simulink model "Solar_position_model"  (R2024a)
settings: Solver=VariableStepAuto  StartTime=0.0  StopTime=5  RelTol=1e-3
Description:
  | Acccurate Solar positioning algorithm
settings Model: Creator=Asus  LastModifiedBy=Asus

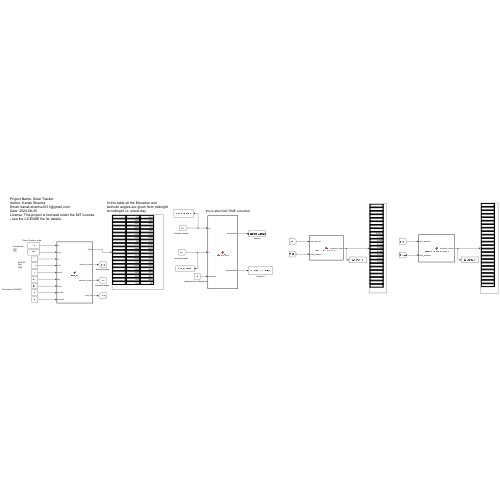
[thumbnail: Simulink's stored preview of the top-level diagram]
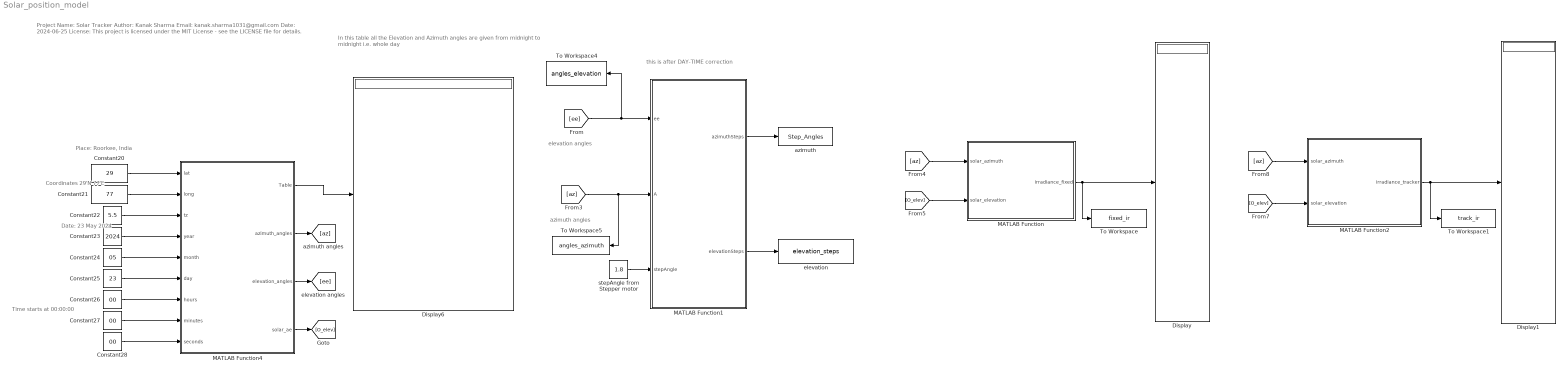
== system Solar_position_model ==
  note: Project Name: Solar Tracker
      | Author: Kanak Sharma
      | Email: kanak.sharma1031@gmail.com
      | Date: 2024-06-25
      | License: This project is licensed under the MIT License - see the LICENSE file for details.
  note: elevation angles
  note: In this table all the Elevation and Azimuth angles are given from midnight to midnight i.e. whole day
  note: Time starts at 00:00:00
  note: Coordinates
      | 29'N
      | 77'E
  note: azimuth angles
  note: this is after DAY-TIME correction
  note: Date: 23 May 2024
  note: Place: Roorkee, India
  Constant20 : Constant  Value=29
  Constant21 : Constant  Value=77
  Constant22 : Constant  Value=5.5
  Constant23 : Constant  Value=2024
  Constant24 : Constant  Value=05
  Constant25 : Constant  Value=23
  Constant26 : Constant  Value=00
  Constant27 : Constant  Value=00
  Constant28 : Constant  Value=00
  Display : Display
  Display1 : Display
  Display6 : Display
  MATLAB Function : MATLAB Function  TreatAsAtomicUnit=on
  MATLAB Function1 : MATLAB Function  TreatAsAtomicUnit=on
  MATLAB Function2 : MATLAB Function  TreatAsAtomicUnit=on
  MATLAB Function4 : MATLAB Function  TreatAsAtomicUnit=on
  To Workspace : ToWorkspace  VariableName=fixed_ir  SampleTime=-1
  To Workspace1 : ToWorkspace  VariableName=track_ir  SampleTime=-1
  To Workspace4 : ToWorkspace  VariableName=angles_elevation  SampleTime=-1
  To Workspace5 : ToWorkspace  VariableName=angles_azimuth  SampleTime=-1
  azimuth : ToWorkspace  VariableName=Step_Angles  SampleTime=-1
  elevation : ToWorkspace  VariableName=elevation_steps  SampleTime=-1
  stepAngle from Stepper motor : Constant  Value=1.8
  wires:
  MATLAB Function4/2(azimuth_angles) -> [az]
  Constant26/1 -> MATLAB Function4/7(hours)
  Constant25/1 -> MATLAB Function4/6(day)
  Constant22/1 -> MATLAB Function4/3(tz)
  MATLAB Function4/3(elevation_angles) -> [ee]
  Constant28/1 -> MATLAB Function4/9(seconds)
  Constant27/1 -> MATLAB Function4/8(minutes)
  MATLAB Function4/1(Table) -> Display6/1
  stepAngle from Stepper motor/1 -> MATLAB Function1/3(stepAngle)
  Constant20/1 -> MATLAB Function4/1(lat)
  MATLAB Function1/2(elevationSteps) -> elevation/1
  Constant21/1 -> MATLAB Function4/2(long)
  [az] -> MATLAB Function1/2(A), To Workspace5/1
  MATLAB Function1/1(azimuthSteps) -> azimuth/1
  [ee] -> MATLAB Function1/1(ee), To Workspace4/1
  Constant24/1 -> MATLAB Function4/5(month)
  MATLAB Function4/4(solar_ae) -> [O_elev]
  Constant23/1 -> MATLAB Function4/4(year)
  MATLAB Function2/1(irradiance_tracker) -> Display1/1, To Workspace1/1
  [O_elev] -> MATLAB Function/2(solar_elevation)
  [az] -> MATLAB Function2/1(solar_azimuth)
  [O_elev] -> MATLAB Function2/2(solar_elevation)
  MATLAB Function/1(irradiance_fixed) -> Display/1, To Workspace/1
  [az] -> MATLAB Function/1(solar_azimuth)

== matlab function Solar_position_model/MATLAB Function1 ==
  data: ee input; azimuthSteps output; A input; stepAngle input; elevationSteps output
%{
Project Name: Solar Tracker
Author: Kanak Sharma
Email: kanak.sharma1031@gmail.com
Date: 2024-06-24
License: This project is licensed under the MIT License - see the LICENSE file for details.
%}
function [azimuthSteps, elevationSteps] = calculateSteps(ee, A, stepAngle)
    % Assuming the stepper motor moves in fixed steps (e.g., 1.8 degrees per step)
    stepAngle;
    
    % Calculate the number of steps required for azimuth
    azimuthSteps = round(A / stepAngle);
    
    % Calculate the number of steps required for elevation
    elevationSteps = round(ee / stepAngle);

 
end

== matlab function Solar_position_model/MATLAB Function ==
  data: solar_azimuth input; irradiance_fixed output; solar_elevation input
function irradiance_fixed = calculate_fixed_irradiance(solar_azimuth, solar_elevation)
    % Fixed panel parameters
    panel_azimuth = 180; % Facing south
    panel_tilt = 15; % Fixed tilt angle

    % Initialize the output
    irradiance_fixed = zeros(1, 24);

    for i = 1:24
        % Calculate irradiance for each hour
        irradiance_fixed(i) = calculate_irradiance(solar_azimuth(i), solar_elevation(i), panel_azimuth, panel_tilt);
    end
end

function irradiance = calculate_irradiance(solar_azimuth, solar_elevation, panel_azimuth, panel_tilt)
    % Check if the solar elevation is below the horizon
    if solar_elevation <= 0
        irradiance = 0;
    else
        % Calculate the cosine of the angle of incidence
        cos_incident_theta = cosd(solar_elevation)*cosd(90-panel_tilt)*cosd(solar_azimuth-panel_azimuth)+sind(solar_elevation)*sind(90-panel_tilt);
        irradiance = max(0, cos_incident_theta);
    end
end

== matlab function Solar_position_model/MATLAB Function2 ==
  data: solar_azimuth input; irradiance_tracker output; solar_elevation input
function irradiance_tracker = calculate_tracker_irradiance(solar_azimuth, solar_elevation)
    % Initialize the output
    irradiance_tracker = zeros(1, 24);

    for i = 1:24
        % Tracker aligns with the sun
        panel_elevation = solar_elevation(i);
        panel_azimuth = solar_azimuth(i);
        
        % Calculate irradiance for each hour
        irradiance_tracker(i) = calculate_irradiance(solar_azimuth(i), solar_elevation(i), panel_azimuth, panel_elevation);
    end
end

function irradiance = calculate_irradiance(solar_azimuth, solar_elevation, panel_azimuth, panel_elevation)
    % Check if the solar elevation is below the horizon
    if solar_elevation < 0
        irradiance = 0;
    else
        % Calculate angle differences
        angle_diff_azimuth = mod(abs(solar_azimuth - panel_azimuth), 360);
        angle_diff_elevation = abs(solar_elevation - panel_elevation);
        
        % Calculate irradiance based on the angle differences
        % Use the angle of incidence (adjusted for panel elevation)
        irradiance = max(0, cosd(angle_diff_azimuth) * cosd(angle_diff_elevation));
    end
end

== matlab function Solar_position_model/MATLAB Function4 ==
  data: lat input; Table output; long input; tz input; year input; month input; day input; hours input; minutes input; seconds input; azimuth_angles output; elevation_angles output; solar_ae output
%{
Project Name: Solar Tracker
Author: Kanak Sharma
Email: kanak.sharma1031@gmail.com
Date: 2024-06-24
License: This project is licensed under the MIT License - see the LICENSE file for details.
%}
function [Table, azimuth_angles, elevation_angles, solar_ae]=solar_ae(lat, long, tz, year, month, day, hours, minutes, seconds)
dd = datetime(year, month, day, hours, minutes, seconds);
n=1;
elevation_angles = zeros(1, 24);
solar_ae = zeros(1,24); solar_ah = zeros(1,24);
Table = zeros(24, 3);
azimuth_angles = zeros(1, 24);

%Reference:
% The NOAA Solar Calculator provides solar position calculations
% based on latitude, longitude, date, and time. These values are 
% essential for determining the optimal positioning of solar panels 
% to maximize energy absorption.
for i = 1:24
    % Calculate e2 as the fraction of the day passed
    e2 = (i-1)/24;
    % Calculate the Julian date
    a = floor((14 - month) / 12);
    y = year + 4800 - a;
    m = month + 12 * a - 3;
    jd = day + floor((153 * m + 2) / 5) + 365 * y + floor(y / 4) - floor(y / 100) + floor(y / 400) - 32045;
    jd = jd + (hours - 12) / 24 + minutes / 1440 + seconds / 86400; 
    julian = jd + e2 - (tz / 24);
    % Calculate Julian century
    julian_cent = (julian - 2451545) / 36525;
    i2 = mod(280.46646 + julian_cent * (36000.76983 + julian_cent * 0.0003032), 360);
    j2 = 357.52911+julian_cent*(35999.05029-0.0001537*julian_cent);
    k2 = 0.016708634 - julian_cent*(0.000042037+0.0000001267*julian_cent);
    % Calculate the sun's equation of the center
    l2 = sin(deg2rad(j2))*(1.914602-julian_cent*(0.004817+0.000014*julian_cent))+sin(deg2rad(2*j2))*(0.019993-0.000101*julian_cent)+sin(deg2rad(3*j2))*0.000289;
    m2=i2+l2;
    n2 = j2 + l2;
    o2 = (1.000001018*(1-k2*k2))/(1+k2*cos(deg2rad(n2)));
    p2 = m2 - 0.00569 - 0.00478 * sin(deg2rad(125.04-1934.136*julian_cent));
    q2 = 23 + (26+((21.448-julian_cent*(46.815+julian_cent*(0.00059-julian_cent*0.001813))))/60)/60;
    r2 = q2+ 0.00256*cos(deg2rad(125.04-1934.136*julian_cent));
    % Calculate the sun's right ascension
    s2 = rad2deg(atan2(cos(deg2rad(p2)),cos(deg2rad(r2))*sin(deg2rad(p2))));
    t2 = rad2deg(asin(sin(deg2rad(r2))*sin(deg2rad(p2))));
    % Calculate the equation of time
    u2 = tan(deg2rad(r2/2))*tan(deg2rad(r2/2));
    v2 = 4*rad2deg(u2*sin(2*deg2rad(i2))-2*k2*sin(deg2rad(j2))+4*k2*u2*sin(deg2rad(j2))*cos(2*deg2rad(i2))-0.5*u2*u2*sin(4*deg2rad(i2))-1.25*k2*k2*sin(2*deg2rad(j2)));
    % Calculate the hour angle of sunrise
    w2 = rad2deg(acos(cos(deg2rad(90.833))/(cos(deg2rad(lat))*cos(deg2rad(t2)))-tan(deg2rad(lat))*tan(deg2rad(t2))));
    x2 = (720-4*lat-v2+tz*60)/1440;
    % Calculate sunrise and sunset times
    y2 = x2-w2*4/1440;
    z2 = x2+w2*4/1440;
    % Calculate the duration of sunlight in minutes
    aa = 8*w2;
    ab = mod(e2*1440+v2+4*long-60*tz,1440);
    ab2 = ab ; 
    %Calculations for Elevation and Azimuth angles
    if ab2 / 4 < 0
        ac = ab2 / 4 + 180;
    else
        ac = ab2 / 4 - 180;
    end
    ad = rad2deg(acos(sin(deg2rad(lat))*sin(deg2rad(t2))+cos(deg2rad(lat))*cos(deg2rad(t2))*cos(deg2rad(ac))));
    %elevation angle 
    ae = 90 - ad;
    elevation_angles(i)=ae;
    if ac > 0
        ah = mod(rad2deg(acos(((sin(deg2rad(lat))*cos(deg2rad(ad)))-sin(deg2rad(t2)))/(cos(deg2rad(lat))*sin(deg2rad(ad)))))+180, 360);
    else
        ah = mod(540 - rad2deg(acos(((sin(deg2rad(lat))*cos(deg2rad(ad)))-sin(deg2rad(t2)))/(cos(deg2rad(lat))*sin(deg2rad(ad))))), 360);
    end

    %azimuth angle
    azimuth_angles(i)=ah;

    %Integration in the format of a Table for Display
    Table(i, 1) = i-1; 
    Table(i, 2) = ae;
    Table(i, 3) = ah; 
    
    solar_ae(i) = ae;
    solar_ah(i) = ah;

    %Changes done for Night time
        if elevation_angles(i) > 0
            elevation_angles(i) = 90-elevation_angles(i); 
        end        

        if elevation_angles(i) <= 0
            azimuth_angles(i) = 0; 
            elevation_angles(i) = 90;
        end

end

end
